simulink model "UDPReceive"  (R2018b)
settings: Solver=FixedStepDiscrete  StartTime=0.0  StopTime=inf  FixedStep=0.01  RelTol=1e-3
libraries: etargetslib x1, dspnetwork x1
settings Model: Creator=lenovo  LastModifiedBy=lenovo

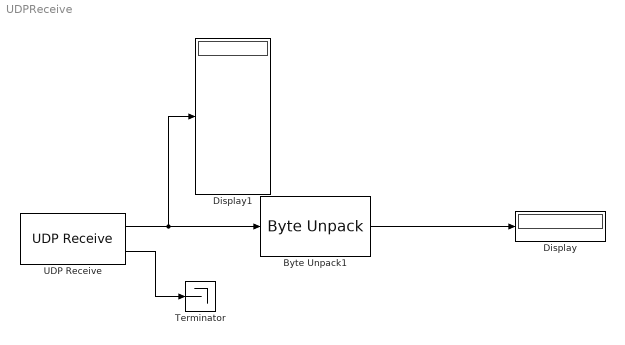
== system UDPReceive ==
  Byte Unpack1 : etargetslib/Byte Unpack  dimensions={[1]}  datatypes={'double'}  byteAlign=1
  Display : Display
  Display1 : Display
  Terminator : Terminator
  UDP Receive : dspnetwork/UDP Receive  localURL='0.0.0.0'  localPort=9090  remoteURL='192.168.71.32'  remotePort=-1  recvBufferSize=8192  dims=8  signalDatatype=uint8  isVarSize=off  showBlockingTime=off  blockingTime=0  sampletime=0.05  blockPlatform=[]
      settings: SourceProductName=DSP System Toolbox  SourceProductBaseCode=DS
  wires:
  UDP Receive/1 -> Byte Unpack1/1, Display1/1
  Byte Unpack1/1 -> Display/1
  UDP Receive/2 -> Terminator/1
